simulink model "task2_lab9"  (R2021a)
settings: Solver=VariableStepAuto  StartTime=0.0  StopTime=10.0  RelTol=1e-3
settings Model: Creator=reemb  LastModifiedBy=reemb

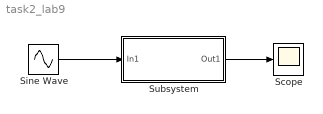
== system task2_lab9 ==
  Scope : Scope
  Sine Wave : Sin  SampleTime=0
  Subsystem : Subsystem  TreatAsAtomicUnit=on  SystemSampleTime=0.5
  wires:
  Sine Wave/1 -> Subsystem/1(In1)
  Subsystem/1(Out1) -> Scope/1

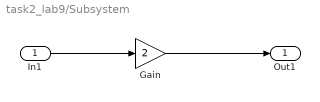
== system task2_lab9/Subsystem ==
  In1 : Inport
  Gain : Gain  Gain=2
  Out1 : Outport
  wires:
  In1/1 -> Gain/1
  Gain/1 -> Out1/1
